simulink model "c_station_v3"  (R2019a)
settings: Solver=VariableStepAuto  StartTime=0.0  StopTime=345600  MaxStep=3600  RelTol=1e-3  AbsTol=1e-3  EnableMultiTasking=on
StopFcn:
  | displayGasParameters(gasPressures);
values from neighbouring files (symbols this model uses):
  conf = gasConfig()    [ColoradoGasModel.m]    (also in gas_v1.m)
  lineParm = [lineParm;add_line("Main 2",24,35,pNom)]    [compressorTest.m]    (also in experiment1.m = [lineParm;add_line("Main 2",24,50,pNom)]; experiment2.m = [lineParm;add_line("Main 3",24,35,pNom)]; experiment3.m = [lineParm;add_line("Aux 3",36,100,pNom)]; experiments12.m)
  loadControlFlag = "on"    [gas_v1.m]
  loadParm = [loadParm; add_load("PP2",pwr,pNom,pCut, stopTime)]    [compressorTest.m]    (also in experiment1.m; experiment2.m; experiment3.m = [loadParm; add_load("PP2",pwr,pNom,pCut,stopTime)]; experiments12.m)
  valveControlFlag = "on"    [ColoradoGasModel.m]    (also in gas_v1.m)
undefined symbols (not defined in the file or in its folder): f, valveParm
libraries: gasLibrary x27, fl_lib x14, nesl_utility x9, instrumentlib x4, SimscapeFluids_lib x1
(part 1 of 3)
settings Model: Creator=dzimm  LastModifiedBy=brandt
settings SolverCC: AutoScaleAbsTol=off
settings DataIOCC: LimitDataPoints=on  MaxDataPoints=10000  ReturnWorkspaceOutputs=off
settings OptimizationCC: LifeSpan=inf
settings DebuggingCC: AllowSymbolicDim=off  PregeneratedLibrarySubsystemCodeDiagnostic=none  SFUnexpectedBacktrackingDiag=warning  SFNoUnconditionalDefaultTransitionDiag=warning  SFExecutionAtInitializationDiag=none  ArithmeticOperatorsInVariantConditions=warning
settings SFSimCC: SimUseLocalCustomCode=off
settings RTWCC: RTWUseLocalCustomCode=off
settings CodeAppCC: StateflowObjectComments=on
settings GRTTargetCC: TargetLangStandard=C89/C90 (ANSI)  GeneratePreprocessorConditionals=Disable all
settings ConfigComp: CovMetricSettings=dw  CovHtmlReporting=on  CovSaveCumulativeToWorkspaceVar=on  CovSaveSingleToWorkspaceVar=on  CovExternalEMLEnable=off  CovSFcnEnable=off
settings SimscapeCC: SimscapeLogType=all  SimscapeLogOpenViewer=on  SimscapeLogLimitData=off  SimscapeLogDataHistory=10000  SimscapeOperatingPoint=op

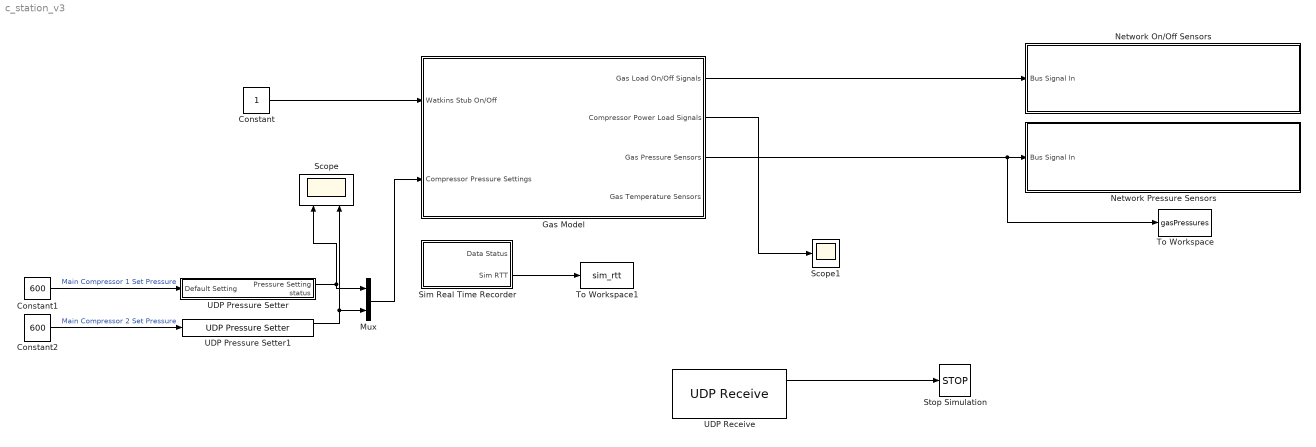
== system c_station_v3 ==
  Constant : Constant
  Constant1 : Constant  Value=600
  Constant2 : Constant  Value=600
  Gas Model : Subsystem
  Mux : Mux  Inputs=2
  Network On/Off Sensors : Subsystem
  Network Pressure Sensors : Subsystem
  Scope : Scope  NumInputPorts=2
  Scope1 : Scope
  Sim Real Time Recorder : Subsystem  AncestorBlock=gasLibrary/Sim Real Time Recorder
  Stop Simulation : Stop
  To Workspace : ToWorkspace  VariableName=gasPressures  SaveFormat=Timeseries  SampleTime=-1
  To Workspace1 : ToWorkspace  VariableName=sim_rtt  SaveFormat=Timeseries  SampleTime=-1
  UDP Pressure Setter : Subsystem  AncestorBlock=gasLibrary/UDP Pressure Setter  mask{LocalPort=6062}
      mask prompts: LocalPort "Local port:"
      mask TypeOptions LocalPort: UDP Receive/LocalPort
  UDP Pressure Setter1 : gasLibrary/UDP Pressure Setter  LocalPort=6063
  UDP Receive : instrumentlib/UDP Receive  Host=localhost  Port=9090  LocalPort=6061  EnablePortSharing=off  GetLatestData=off  DataSize=[1 1]  DataType=double  ASCIIFormatting=%f,  Terminator=LF  ByteOrder=BigEndian  EnableBlockingMode=off  Timeout=10  SampleTime=300  LocalAddress=localhost
      settings: SourceProductName=Instrument Control Toolbox
  wires:
  Constant/1 -> Gas Model/1(Watkins Stub On/Off)
  Mux/1 -> Gas Model/2(Compressor Pressure Settings)
  Gas Model/3(Gas Pressure Sensors) -> Network Pressure Sensors/1(Bus Signal In), To Workspace/1
  Gas Model/1(Gas Load On/Off Signals) -> Network On/Off Sensors/1(Bus Signal In)
  Sim Real Time Recorder/2(Sim RTT) -> To Workspace1/1
  UDP Receive/1 -> Stop Simulation/1
  Constant1/1 -> UDP Pressure Setter/1(Default Setting)  "Main Compressor 1 Set Pressure"
  UDP Pressure Setter/1("Pressure Setting ") -> Mux/1, Scope/1
  UDP Pressure Setter1/1 -> Scope/2, Mux/2
  Constant2/1 -> UDP Pressure Setter1/1  "Main Compressor 2 Set Pressure"
  Gas Model/2("Compressor Power Load Signals ") -> Scope1/1
